simulink model "Tuning_PID"  (R2019b)
settings: Solver=VariableStepAuto  StartTime=0.0  StopTime=150  RelTol=1e-3
undefined symbols (not defined in the file or in its folder): k
settings Model: Creator=Rami  LastModifiedBy=Rami
settings SolverCC: MaxConsecutiveZCs=10000  MaxConsecutiveMinStep=1000
settings DataIOCC: ReturnWorkspaceOutputs=off

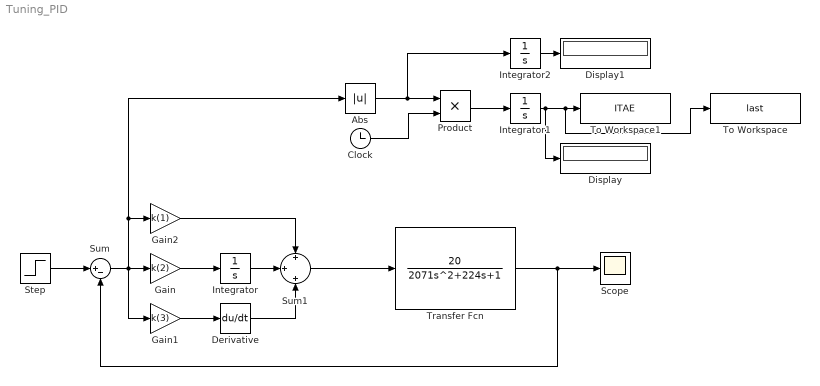
== system Tuning_PID ==
  Abs : Abs
  Clock : Clock
  Derivative : Derivative
  Display : Display
  Display1 : Display
  Gain : Gain  Gain=k(2)
  Gain1 : Gain  Gain=k(3)
  Gain2 : Gain  Gain=k(1)
  Integrator : Integrator
  Integrator1 : Integrator
  Integrator2 : Integrator
  Product : Product
  Scope : Scope
  Step : Step  SampleTime=0
  Sum : Sum  Inputs=|+-
  Sum1 : Sum  Inputs=+|+|+
  To Workspace : ToWorkspace  VariableName=last  SampleTime=-1
      settings: MaxDataPoints=1
  To Workspace1 : ToWorkspace  VariableName=ITAE  SampleTime=-1
  Transfer Fcn : TransferFcn  Numerator=[20]  Denominator=[2071 224 1]
  wires:
  Transfer Fcn/1 -> Scope/1, Sum/2
  Sum/1 -> Gain1/1, Gain/1, Abs/1, Gain2/1
  Gain2/1 -> Sum1/1
  Gain/1 -> Integrator/1
  Integrator/1 -> Sum1/2
  Gain1/1 -> Derivative/1
  Derivative/1 -> Sum1/3
  Sum1/1 -> Transfer Fcn/1
  Step/1 -> Sum/1
  Abs/1 -> Integrator2/1, Product/1
  Clock/1 -> Product/2
  Product/1 -> Integrator1/1
  Integrator1/1 -> To Workspace/1, To Workspace1/1, Display/1
  Integrator2/1 -> Display1/1
